simulink model "Go_discreta"  (Simulink 5.0)
settings: Solver=ode45  StartTime=0.0  StopTime=10.0  RelTol=1e-3
undefined symbols (not defined in the file): a, d, q, Vd
libraries: dspsigops x1
settings Model: LastModifiedBy=pc1

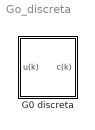
== system Go_discreta ==
  G0 discreta : Subsystem

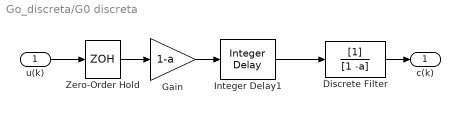
== system Go_discreta/G0 discreta ==
  u(k) : Inport
  Discrete Filter : DiscreteFilter  Denominator=[1 -a]  SampleTime=Vd/(d*q)
  Gain : Gain  Gain=1-a  SaturateOnIntegerOverflow=on
  Integer Delay1 : dspsigops/Integer Delay  delay=d+1  ic=0.5  reset_popup=None
  Zero-Order Hold : ZeroOrderHold  SampleTime=Vd/(d*q)
  c(k) : Outport
  wires:
  Zero-Order Hold/1 -> Gain/1
  Gain/1 -> Integer Delay1/1
  Integer Delay1/1 -> Discrete Filter/1
  Discrete Filter/1 -> c(k)/1
  u(k)/1 -> Zero-Order Hold/1
